simulink library "DFIM_Tutorial_Library"  (R2019b)
settings: Solver=VariableStepAuto  StartTime=0.0  StopTime=10.0  RelTol=1e-3
values from neighbouring files (symbols this model uses):
  f = 50    [init.m]
  Fs = Vs * sqrt(2/3)/(2*pi*f)    [init.m]
  Lg = 400e-6    (= 0.0004)    [init.m]
  Lr = Lm + Lsi    (= 0.002587)    [init.m]
  N = 100    [init.m]
  p = 2    [init.m]
  Rayon = 42    [init.m]
  ro = 1.225    [init.m]
  sigma = 1 - Lm^2/(Ls*Lr)    (= 0.0661284179513)    [init.m]
  tab_lambda = [0.1:0.01:11.8]    [init.m]
undefined symbols (not defined in the file or in its folder): Ct, DiscIntNeverNeededParam
settings Model: Creator=anony  LastModifiedBy=anony

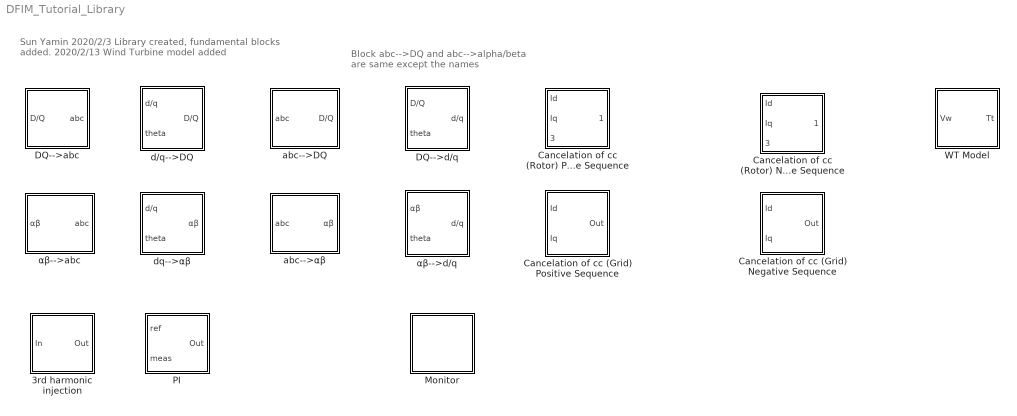
== system DFIM_Tutorial_Library ==
  note: Block abc-->DQ and abc-->alpha/beta
      | are same except the names
  note: Sun Yamin
      | 2020/2/3 Library created, fundamental blocks added.
      | 2020/2/13 Wind Turbine model added
  3rd harmonic injection : Subsystem
  Cancelation of cc (Grid) Negative Sequence : Subsystem
  Cancelation of cc (Grid) Positive Sequence : Subsystem
  Cancelation of cc (Rotor) Negative Sequence : Subsystem
  Cancelation of cc (Rotor) Positive Sequence : Subsystem
  DQ-->abc : Subsystem
  DQ-->d/q : Subsystem
  Monitor : Subsystem
  PI : Subsystem  mask{kp=1, ki=1, int_uppper_limit=inf, int_lower_limit=-inf, total_upper_limit=inf, total_lower_limit=-inf, sample_time=-1}
      mask prompts: kp "Proportion Gain"; ki "Integrator Gain"; int_uppper_limit "Integrator Upper Limit"; int_lower_limit "Integrator Lower Limit"; total_upper_limit "Total Upper Limit"; total_lower_limit "Total Lower Limit"; sample_time "Sample Time"
  WT Model : Subsystem
  abc-->DQ : Subsystem
  abc-->αβ : Subsystem
  d/q-->DQ : Subsystem
  dq-->αβ : Subsystem
  αβ-->abc : Subsystem
  αβ-->d/q : Subsystem

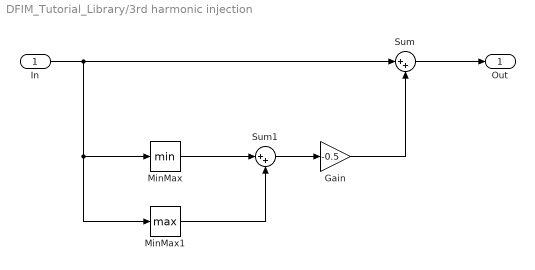
== system DFIM_Tutorial_Library/3rd harmonic injection ==
  In : Inport
  Gain : Gain  Gain=-0.5
  MinMax : MinMax
  MinMax1 : MinMax  Function=max
  Sum : Sum  Inputs=|++
  Sum1 : Sum  Inputs=|++
  Out : Outport
  wires:
  In/1 -> MinMax1/1, MinMax/1, Sum/1
  MinMax/1 -> Sum1/1
  MinMax1/1 -> Sum1/2
  Gain/1 -> Sum/2
  Sum1/1 -> Gain/1
  Sum/1 -> Out/1

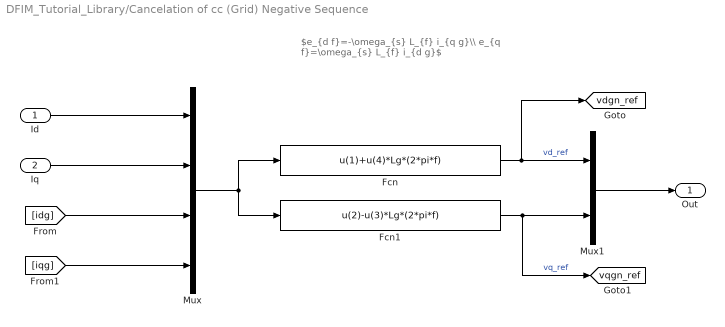
== system DFIM_Tutorial_Library/Cancelation of cc (Grid) Negative Sequence ==
  note: $e_{d f}=-\omega_{s} L_{f} i_{q g}\\ e_{q f}=\omega_{s} L_{f} i_{d g}$
  Id : Inport
  Iq : Inport  Port=2
  Fcn : Fcn  Expr=u(1)+u(4)*Lg*(2*pi*f)
  Fcn1 : Fcn  Expr=u(2)-u(3)*Lg*(2*pi*f)
  Mux : Mux
  Mux1 : Mux  Inputs=2
  Out : Outport
  tag scope: vdgn_ref=global, vqgn_ref=global
  wires:
  Fcn1/1 -> [vqgn_ref], Mux1/2  "vq_ref"
  Id/1 -> Mux/1
  Mux/1 -> Fcn1/1, Fcn/1
  [idg] -> Mux/3
  Mux1/1 -> Out/1
  [iqg] -> Mux/4
  Iq/1 -> Mux/2
  Fcn/1 -> [vdgn_ref], Mux1/1  "vd_ref"

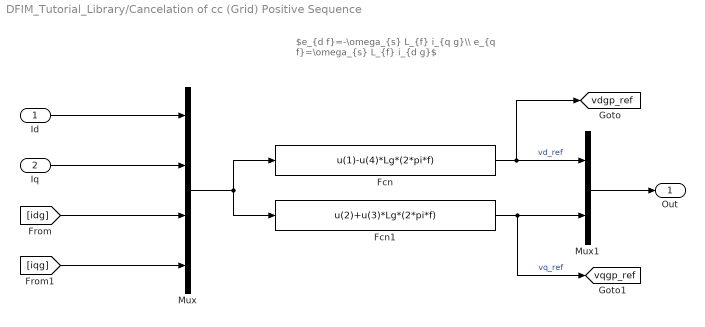
== system DFIM_Tutorial_Library/Cancelation of cc (Grid) Positive Sequence ==
  note: $e_{d f}=-\omega_{s} L_{f} i_{q g}\\ e_{q f}=\omega_{s} L_{f} i_{d g}$
  Id : Inport
  Iq : Inport  Port=2
  Fcn : Fcn  Expr=u(1)-u(4)*Lg*(2*pi*f)
  Fcn1 : Fcn  Expr=u(2)+u(3)*Lg*(2*pi*f)
  Mux : Mux
  Mux1 : Mux  Inputs=2
  Out : Outport
  tag scope: vdgp_ref=global, vqgp_ref=global
  wires:
  Mux1/1 -> Out/1
  Iq/1 -> Mux/2
  [idg] -> Mux/3
  [iqg] -> Mux/4
  Mux/1 -> Fcn1/1, Fcn/1
  Fcn/1 -> [vdgp_ref], Mux1/1  "vd_ref"
  Fcn1/1 -> [vqgp_ref], Mux1/2  "vq_ref"
  Id/1 -> Mux/1

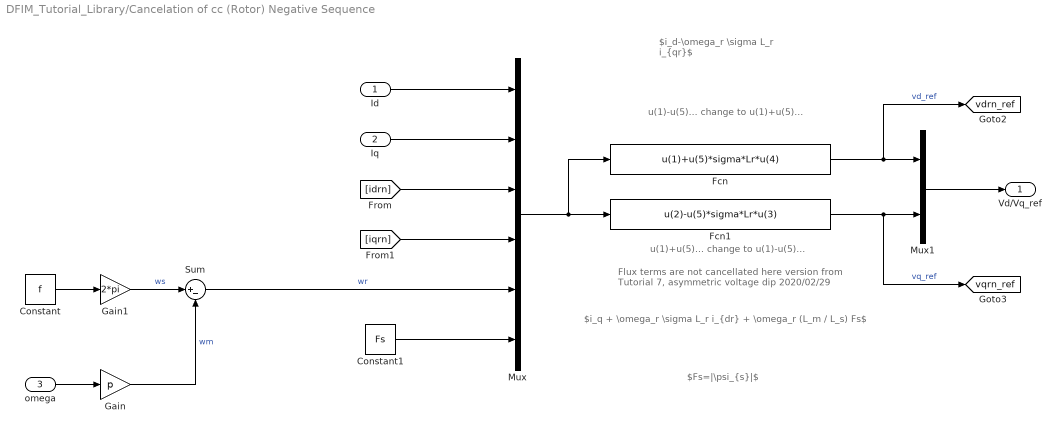
== system DFIM_Tutorial_Library/Cancelation of cc (Rotor) Negative Sequence ==
  note: u(1)-u(5)... change to u(1)+u(5)...
  note: $i_d-\omega_r \sigma L_r i_{qr}$
  note: $i_q + \omega_r \sigma L_r i_{dr} + \omega_r (L_m / L_s) Fs$
  note: Flux terms are not cancellated here
      | version from Tutorial 7, asymmetric voltage dip
      | 2020/02/29
  note: $Fs=|\psi_{s}|$
  note: u(1)+u(5)... change to u(1)-u(5)...
  Id : Inport
  Iq : Inport  Port=2
  omega : Inport  Port=3
  Constant : Constant  Value=f
  Constant1 : Constant  Value=Fs
  Fcn : Fcn  Expr=u(1)+u(5)*sigma*Lr*u(4)
  Fcn1 : Fcn  Expr=u(2)-u(5)*sigma*Lr*u(3)
  Gain : Gain  Gain=p
  Gain1 : Gain  Gain=2*pi
  Mux : Mux  Inputs=6
  Mux1 : Mux  Inputs=2
  Sum : Sum  Inputs=|+-
  Vd/Vq_ref : Outport
  tag scope: vdrn_ref=global, vqrn_ref=global
  wires:
  Id/1 -> Mux/1
  [iqrn] -> Mux/4
  Iq/1 -> Mux/2
  Mux/1 -> Fcn/1, Fcn1/1
  [idrn] -> Mux/3
  Fcn/1 -> [vdrn_ref], Mux1/1  "vd_ref"
  Fcn1/1 -> [vqrn_ref], Mux1/2  "vq_ref"
  Mux1/1 -> Vd/Vq_ref/1
  Gain1/1 -> Sum/1  "ws"
  Constant/1 -> Gain1/1
  Sum/1 -> Mux/5  "wr"
  Gain/1 -> Sum/2  "wm"
  omega/1 -> Gain/1
  Constant1/1 -> Mux/6

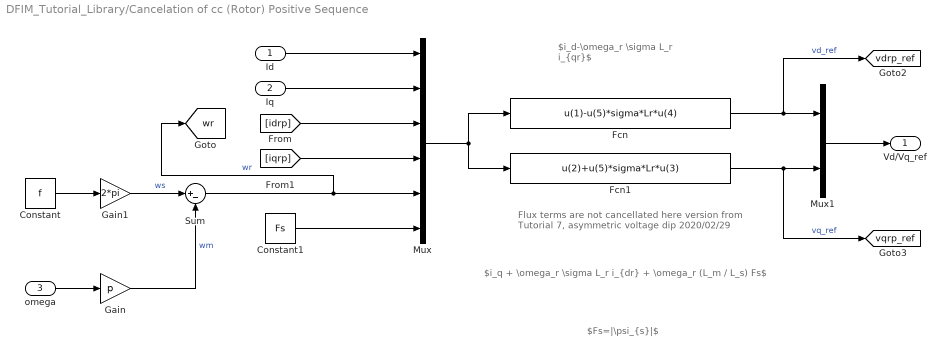
== system DFIM_Tutorial_Library/Cancelation of cc (Rotor) Positive Sequence ==
  note: Flux terms are not cancellated here
      | version from Tutorial 7, asymmetric voltage dip
      | 2020/02/29
  note: $Fs=|\psi_{s}|$
  note: $i_d-\omega_r \sigma L_r i_{qr}$
  note: $i_q + \omega_r \sigma L_r i_{dr} + \omega_r (L_m / L_s) Fs$
  Id : Inport
  Iq : Inport  Port=2
  omega : Inport  Port=3
  Constant : Constant  Value=f
  Constant1 : Constant  Value=Fs
  Fcn : Fcn  Expr=u(1)-u(5)*sigma*Lr*u(4)
  Fcn1 : Fcn  Expr=u(2)+u(5)*sigma*Lr*u(3)
  Gain : Gain  Gain=p
  Gain1 : Gain  Gain=2*pi
  Mux : Mux  Inputs=6
  Mux1 : Mux  Inputs=2
  Sum : Sum  Inputs=|+-
  Vd/Vq_ref : Outport
  tag scope: vdrp_ref=global, vqrp_ref=global, wr=global
  wires:
  Constant/1 -> Gain1/1
  Gain1/1 -> Sum/1  "ws"
  Gain/1 -> Sum/2  "wm"
  omega/1 -> Gain/1
  Id/1 -> Mux/1
  Iq/1 -> Mux/2
  [idrp] -> Mux/3
  [iqrp] -> Mux/4
  Sum/1 -> [wr], Mux/5  "wr"
  Constant1/1 -> Mux/6
  Fcn/1 -> [vdrp_ref], Mux1/1  "vd_ref"
  Fcn1/1 -> [vqrp_ref], Mux1/2  "vq_ref"
  Mux/1 -> Fcn/1, Fcn1/1
  Mux1/1 -> Vd/Vq_ref/1

== system DFIM_Tutorial_Library/DQ-->abc ==
  note: $\left[\begin{array}{c} {x_{a}} \\ {x_{b}} \\ {x_{c}} \end{array}\right]=\left[\begin{array}{cc} {1} & {0} \\ {-\frac{1}{2}} & {\frac{\sqrt{3}}{2}} \\ {-\frac{1}{2}} & {-\frac{\sqrt{3}}{2}} \end{array}\right]\left[\begin{array}{c} {x_{\alpha}} \\ {x_{\beta}} \end{array}\right]$
  D/Q : Inport
  Fcn : Fcn  Expr=u(1)
  Fcn1 : Fcn  Expr=-(u(1))/2 + (u(2)*sqrt(3)/2)
  Fcn2 : Fcn  Expr=-(u(1)/2) - u(2)*(sqrt(3)/2)
  Mux : Mux  Inputs=3
  abc : Outport
  wires:
  Fcn/1 -> Mux/1
  Fcn1/1 -> Mux/2
  Fcn2/1 -> Mux/3
  Mux/1 -> abc/1
  D/Q/1 -> Fcn2/1, Fcn/1, Fcn1/1

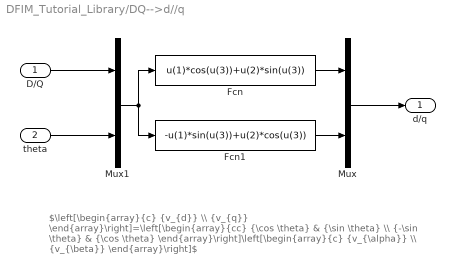
== system DFIM_Tutorial_Library/DQ-->d//q ==
  note: $\left[\begin{array}{c} {v_{d}} \\ {v_{q}} \end{array}\right]=\left[\begin{array}{cc} {\cos \theta} & {\sin \theta} \\ {-\sin \theta} & {\cos \theta} \end{array}\right]\left[\begin{array}{c} {v_{\alpha}} \\ {v_{\beta}} \end{array}\right]$
  D/Q : Inport
  theta : Inport  Port=2
  Fcn : Fcn  Expr=u(1)*cos(u(3))+u(2)*sin(u(3))
  Fcn1 : Fcn  Expr=-u(1)*sin(u(3))+u(2)*cos(u(3))
  Mux : Mux  Inputs=2
  Mux1 : Mux  Inputs=2
  d/q : Outport
  wires:
  Fcn1/1 -> Mux/2
  Mux/1 -> d/q/1
  Fcn/1 -> Mux/1
  Mux1/1 -> Fcn1/1, Fcn/1
  D/Q/1 -> Mux1/1
  theta/1 -> Mux1/2

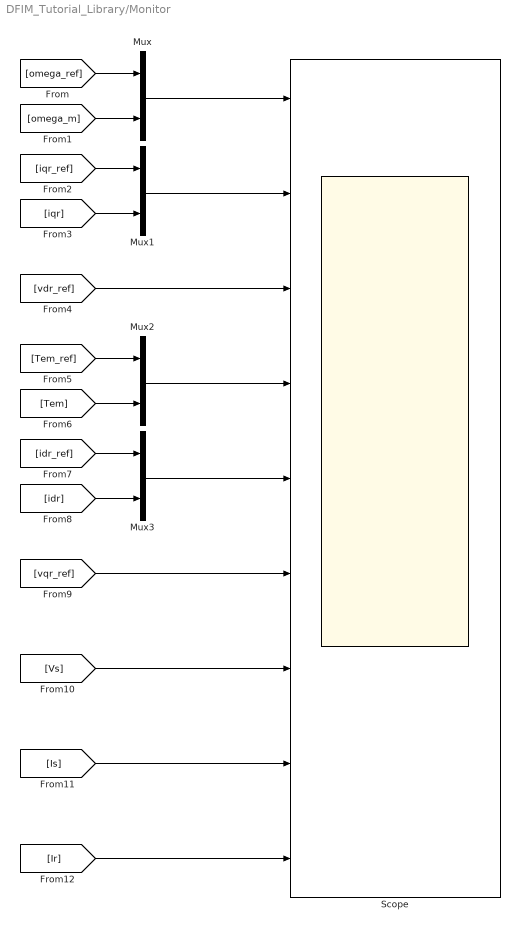
== system DFIM_Tutorial_Library/Monitor ==
  Mux{,1..3} (4 alike) : Mux  Inputs=2
  Scope : Scope  NumInputPorts=9
  wires:
  [omega_ref] -> Mux/1
  [omega_m] -> Mux/2
  [iqr_ref] -> Mux1/1
  [iqr] -> Mux1/2
  [Tem_ref] -> Mux2/1
  [Tem] -> Mux2/2
  [idr_ref] -> Mux3/1
  [idr] -> Mux3/2
  Mux/1 -> Scope/1
  Mux1/1 -> Scope/2
  [vdr_ref] -> Scope/3
  Mux2/1 -> Scope/4
  Mux3/1 -> Scope/5
  [vqr_ref] -> Scope/6
  [Vs] -> Scope/7
  [Is] -> Scope/8
  [Ir] -> Scope/9

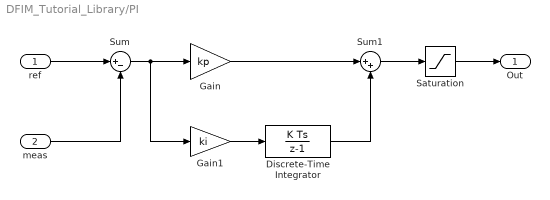
== system DFIM_Tutorial_Library/PI ==
  ref : Inport
  meas : Inport  Port=2
  Discrete-Time Integrator : DiscreteIntegrator  SampleTime=sample_time  LimitOutput=on  UpperSaturationLimit=int_uppper_limit  LowerSaturationLimit=int_lower_limit  ICPrevOutput=DiscIntNeverNeededParam  ICPrevScaledInput=DiscIntNeverNeededParam
  Gain : Gain  Gain=kp
  Gain1 : Gain  Gain=ki
  Saturation : Saturate  UpperLimit=total_upper_limit  LowerLimit=total_lower_limit
  Sum : Sum  Inputs=|+-
  Sum1 : Sum  Inputs=|++
  Out : Outport
  wires:
  ref/1 -> Sum/1
  Gain1/1 -> Discrete-Time Integrator/1
  Sum1/1 -> Saturation/1
  Saturation/1 -> Out/1
  Sum/1 -> Gain1/1, Gain/1
  Gain/1 -> Sum1/1
  Discrete-Time Integrator/1 -> Sum1/2
  meas/1 -> Sum/2

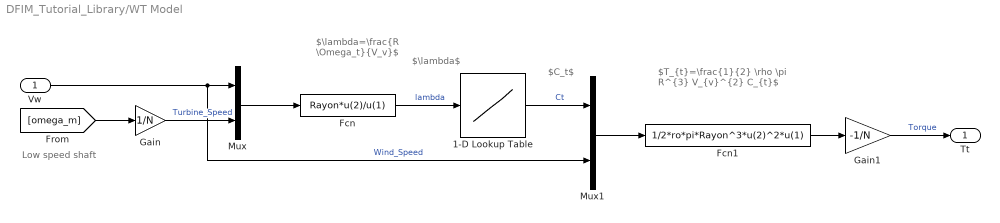
== system DFIM_Tutorial_Library/WT Model ==
  note: Low speed shaft
  note: $T_{t}=\frac{1}{2} \rho \pi R^{3} V_{v}^{2} C_{t}$
  note: $\lambda=\frac{R \Omega_t}{V_v}$
  note: $C_t$
  note: $\lambda$
  Vw : Inport
  1-D Lookup Table : Lookup_n-D  NumberOfTableDimensions=1  BreakpointsForDimension1=tab_lambda  Table=Ct  InternalRulePriority=Speed  RndMeth=Simplest  InputSameDT=on
  Fcn : Fcn  Expr=Rayon*u(2)/u(1)
  Fcn1 : Fcn  Expr=1/2*ro*pi*Rayon^3*u(2)^2*u(1)
  Gain : Gain  Gain=1/N
  Gain1 : Gain  Gain=-1/N
  Mux : Mux  Inputs=2
  Mux1 : Mux  Inputs=2
  Tt : Outport
  wires:
  Mux/1 -> Fcn/1
  Fcn/1 -> 1-D Lookup Table/1  "lambda"
  Gain/1 -> Mux/2  "Turbine_Speed"
  [omega_m] -> Gain/1
  Vw/1 -> Mux1/2, Mux/1  "Wind_Speed"
  1-D Lookup Table/1 -> Mux1/1  "Ct"
  Mux1/1 -> Fcn1/1
  Fcn1/1 -> Gain1/1
  Gain1/1 -> Tt/1  "Torque"

== system DFIM_Tutorial_Library/abc-->DQ ==
  note: $\left[\begin{array}{l} {x_{\alpha}} \\ {x_{\beta}} \end{array}\right]=\frac{2}{3} \cdot\left[\begin{array}{ccc} {1} & {-\frac{1}{2}} & {-\frac{1}{2}} \\ {0} & {\frac{\sqrt{3}}{2}} & {-\frac{\sqrt{3}}{2}} \end{array}\right] \cdot\left[\begin{array}{c} {x_{a}} \\ {x_{b}} \\ {x_{c}} \end{array}\right]$
  abc : Inport
  Fcn : Fcn  Expr=(2/3)*( u(1) - u(2)/2 - u(3)/2 )
  Fcn1 : Fcn  Expr=(2/3) * ( u(2)*(sqrt(3)/2) - u(3)*(sqrt(3)/2) )
  Mux : Mux  Inputs=2
  D/Q : Outport
  wires:
  abc/1 -> Fcn/1, Fcn1/1
  Fcn/1 -> Mux/1
  Fcn1/1 -> Mux/2
  Mux/1 -> D/Q/1

== system DFIM_Tutorial_Library/abc-->αβ ==
  note: $\left[\begin{array}{l} {x_{\alpha}} \\ {x_{\beta}} \end{array}\right]=\frac{2}{3} \cdot\left[\begin{array}{ccc} {1} & {-\frac{1}{2}} & {-\frac{1}{2}} \\ {0} & {\frac{\sqrt{3}}{2}} & {-\frac{\sqrt{3}}{2}} \end{array}\right] \cdot\left[\begin{array}{c} {x_{a}} \\ {x_{b}} \\ {x_{c}} \end{array}\right]$
  abc : Inport
  Fcn : Fcn  Expr=(2/3)*( u(1) - u(2)/2 - u(3)/2 )
  Fcn1 : Fcn  Expr=(2/3) * ( u(2)*(sqrt(3)/2) - u(3)*(sqrt(3)/2) )
  Mux : Mux  Inputs=2
  αβ : Outport
  wires:
  Fcn1/1 -> Mux/2
  abc/1 -> Fcn/1, Fcn1/1
  Fcn/1 -> Mux/1
  Mux/1 -> αβ/1

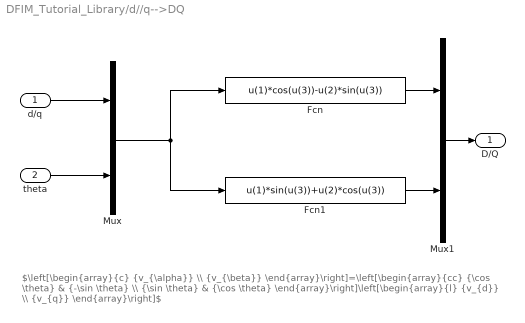
== system DFIM_Tutorial_Library/d//q-->DQ ==
  note: $\left[\begin{array}{c} {v_{\alpha}} \\ {v_{\beta}} \end{array}\right]=\left[\begin{array}{cc} {\cos \theta} & {-\sin \theta} \\ {\sin \theta} & {\cos \theta} \end{array}\right]\left[\begin{array}{l} {v_{d}} \\ {v_{q}} \end{array}\right]$
  d/q : Inport
  theta : Inport  Port=2
  Fcn : Fcn  Expr=u(1)*cos(u(3))-u(2)*sin(u(3))
  Fcn1 : Fcn  Expr=u(1)*sin(u(3))+u(2)*cos(u(3))
  Mux : Mux  Inputs=2
  Mux1 : Mux  Inputs=2
  D/Q : Outport
  wires:
  theta/1 -> Mux/2
  d/q/1 -> Mux/1
  Mux/1 -> Fcn/1, Fcn1/1
  Fcn1/1 -> Mux1/2
  Fcn/1 -> Mux1/1
  Mux1/1 -> D/Q/1

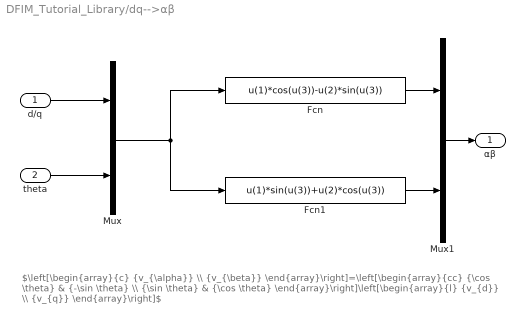
== system DFIM_Tutorial_Library/dq-->αβ ==
  note: $\left[\begin{array}{c} {v_{\alpha}} \\ {v_{\beta}} \end{array}\right]=\left[\begin{array}{cc} {\cos \theta} & {-\sin \theta} \\ {\sin \theta} & {\cos \theta} \end{array}\right]\left[\begin{array}{l} {v_{d}} \\ {v_{q}} \end{array}\right]$
  d/q : Inport
  theta : Inport  Port=2
  Fcn : Fcn  Expr=u(1)*cos(u(3))-u(2)*sin(u(3))
  Fcn1 : Fcn  Expr=u(1)*sin(u(3))+u(2)*cos(u(3))
  Mux : Mux  Inputs=2
  Mux1 : Mux  Inputs=2
  αβ : Outport
  wires:
  d/q/1 -> Mux/1
  Fcn1/1 -> Mux1/2
  Mux1/1 -> αβ/1
  Mux/1 -> Fcn/1, Fcn1/1
  theta/1 -> Mux/2
  Fcn/1 -> Mux1/1

== system DFIM_Tutorial_Library/αβ-->abc ==
  note: $\left[\begin{array}{c} {x_{a}} \\ {x_{b}} \\ {x_{c}} \end{array}\right]=\left[\begin{array}{cc} {1} & {0} \\ {-\frac{1}{2}} & {\frac{\sqrt{3}}{2}} \\ {-\frac{1}{2}} & {-\frac{\sqrt{3}}{2}} \end{array}\right]\left[\begin{array}{c} {x_{\alpha}} \\ {x_{\beta}} \end{array}\right]$
  αβ : Inport
  Fcn : Fcn  Expr=u(1)
  Fcn1 : Fcn  Expr=-(u(1))/2 + (u(2)*sqrt(3)/2)
  Fcn2 : Fcn  Expr=-(u(1)/2) - u(2)*(sqrt(3)/2)
  Mux : Mux  Inputs=3
  abc : Outport
  wires:
  Mux/1 -> abc/1
  Fcn/1 -> Mux/1
  Fcn2/1 -> Mux/3
  αβ/1 -> Fcn2/1, Fcn/1, Fcn1/1
  Fcn1/1 -> Mux/2

== system DFIM_Tutorial_Library/αβ-->d//q ==
  note: $\left[\begin{array}{c} {v_{d}} \\ {v_{q}} \end{array}\right]=\left[\begin{array}{cc} {\cos \theta} & {\sin \theta} \\ {-\sin \theta} & {\cos \theta} \end{array}\right]\left[\begin{array}{c} {v_{\alpha}} \\ {v_{\beta}} \end{array}\right]$
  αβ : Inport
  theta : Inport  Port=2
  Fcn : Fcn  Expr=u(1)*cos(u(3))+u(2)*sin(u(3))
  Fcn1 : Fcn  Expr=-u(1)*sin(u(3))+u(2)*cos(u(3))
  Mux : Mux  Inputs=2
  Mux1 : Mux  Inputs=2
  d/q : Outport
  wires:
  theta/1 -> Mux1/2
  Mux1/1 -> Fcn1/1, Fcn/1
  Fcn1/1 -> Mux/2
  Mux/1 -> d/q/1
  αβ/1 -> Mux1/1
  Fcn/1 -> Mux/1
